simulink model "Q9_simulation"  (R2017b)
settings: Solver=VariableStepAuto  StartTime=0.0  StopTime=10.0  RelTol=1e-3
settings Model: Creator=HeMaTshop  LastModifiedBy=HeMaTshop

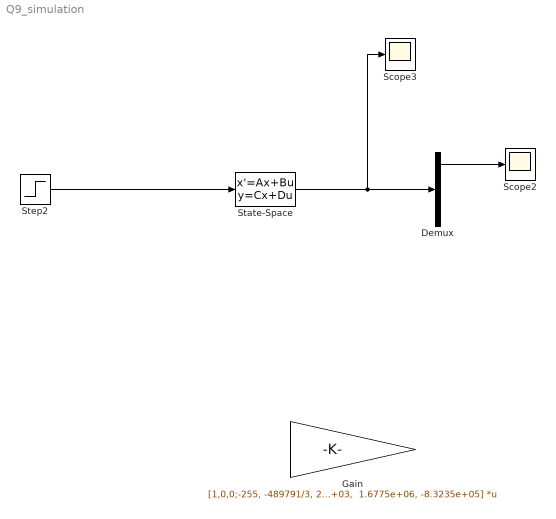
== system Q9_simulation ==
  Demux : Demux  Outputs=3
  Gain : Gain  Gain="[1,0,0;-255, -489791/3, 243470/3;2.5637e+03,  1.6775e+06, -8.3235e+05]"  Multiplication=Matrix(K*u)
  Scope2 : Scope
  Scope3 : Scope
  State-Space : StateSpace  A=[1,2;3,4]  B=[0.0016; 0.0033]  C=eye(2)  D=[1;2]  InitialCondition=0
  Step2 : Step  Time=0  SampleTime=0
  wires:
  Step2/1 -> State-Space/1
  State-Space/1 -> Scope3/1, Demux/1
  Demux/1 -> Scope2/1
